simulink model "MassflowModel"  (R2020b)
settings: Solver=VariableStepAuto  StartTime=0.0  StopTime=55.357742309570312  RelTol=1e-3  AbsTol=1e-3
values from neighbouring files (symbols this model uses):
  coil_specific_heat_transfer = 20    [LoadDataForParameterEstimation.m]
  coil_voltage = 20    [LoadDataForParameterEstimation.m]
libraries: fl_lib x13, nesl_utility x10, SimscapeFluids_lib x1, SignalEditorBlockLib x1
(part 1 of 3)
settings Model: OrderedModelArguments=off  Creator=gam19  LastModifiedBy=gianandrea
settings SolverCC: AutoScaleAbsTol=off
settings DataIOCC: SaveOutput=off  SignalLogging=off  DSMLogging=off  SaveTime=off  ReturnWorkspaceOutputs=off  OutputTimes='[]'  ReturnWorkspaceOutputsName=SDOSimTest_Log
settings DebuggingCC: SymbolicDimsDataTypeCodeGenerationDiagnostic=none
settings SFSimCC: CustomCodeUndefinedFunction=UseInterfaceOnly
settings SimscapeCC: SimscapeLogType=all  SimscapeLogSimulationStatistics=on  SimscapeLogDataHistory=10000

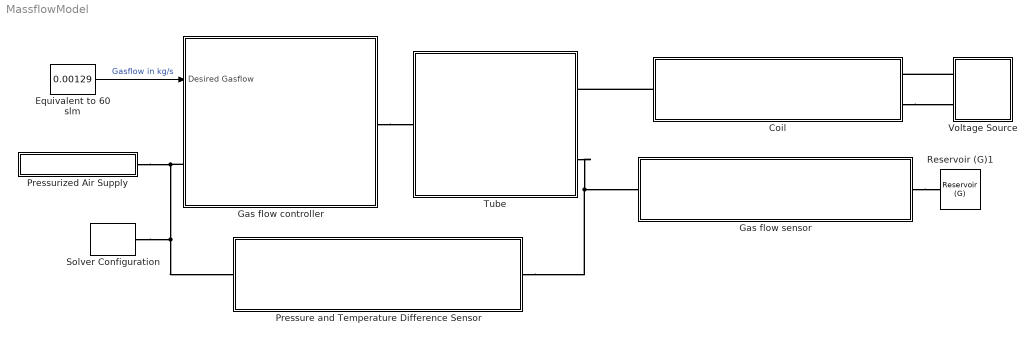
== system MassflowModel ==
  Coil : Subsystem
  Equivalent to 60 slm : Constant  Value=0.00129
  Gas flow controller : Subsystem
  Gas flow sensor : Subsystem
  Pressure and Temperature Difference Sensor : Subsystem
  Pressurized Air Supply : Subsystem
  Reservoir (G)1 : fl_lib/Gas/Elements/Reservoir (G)  pressure_spec=foundation.enum.pressure_spec.atmospheric  reservoir_pressure=0.101325 MPa  reservoir_temperature=300 K  area_A=0.01 m^2
      settings: SourceProductBaseCode=SS
  Solver Configuration : nesl_utility/Solver Configuration  PhysicalDomain=network_engine_domain  SubClassName=solver  LeftPortType=input  RightPortType=generic  Tones=[]  Harmonics=[]  SimulateNoise=off  Profile=off  UseLocalSampling=off  EnableSwitchedLinearOptims=on  FrequencyDomain=off  UseCCode=off  RelTol=0.001  AbsTol=1e-06  MinStep=1e-09  ToWorkspace=off  RevertToSquareIcSolve=off  NumHomotopyIterations=100  PhasorMode=off  PhasorModeNumHarmonics=1  DoDC=off  ResidualTolerance=1e-09  UseLocalSolver=off  LocalSolverChoice=NE_BACKWARD_EULER_ADVANCER  LocalSolverSampleTime=0.001  DoFixedCost=off  MaxNonlinIter=3  MaxModeIter=2  ComputeImpulses=off  ImpulseIterations=2  LinearAlgebra=auto  EquationFormulation=NE_TIME_EF  DelaysMemoryBudget=1024  AutomaticFiltering=on  FilteringTimeConstant=0.001  PartitionStorageMethod=AS_NEEDED  PartitionMemoryBudget=1024  PartitionMethod=ROBUST
  Tube : Subsystem
  Voltage Source : Subsystem
  wires:
  Equivalent to 60 slm/1 -> Gas flow controller/1(Desired Gasflow)  "Gasflow in kg/s"
  connections:
  Pressurized Air Supply/RConn1 -- Pressure and Temperature Difference Sensor/LConn1 -- Solver Configuration/RConn1 -- Gas flow controller/LConn1
  Gas flow controller/RConn1 -- Tube/LConn1
  Coil/LConn1 -- Tube/RConn1
  Tube/RConn2 -- Pressure and Temperature Difference Sensor/RConn1 -- Gas flow sensor/LConn1
  Gas flow sensor/RConn1 -- Reservoir (G)1/LConn1
  Voltage Source/LConn1 -- Coil/RConn1
  Coil/RConn2 -- Voltage Source/LConn2

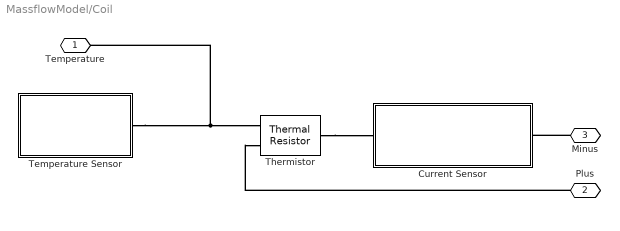
== system MassflowModel/Coil ==
  Current Sensor : Subsystem
  Temperature Sensor : Subsystem
  Thermistor : fl_lib/Electrical/Electrical Elements/Thermal Resistor  R0=9.5 Ohm  T0=298.15 K  alpha=50e-8 1/K  tc=coil_thermal_timeconstant s  K_d=0.0001 W/K  T_specify=off  T_priority=High  T=300 K  T_nominal_specify=off  T_nominal_unit=K  T_nominal_value=1
      settings: SourceProductBaseCode=SS  InternalSimscapePortConfiguration="{\"Bottom\":[],\"Left\":[{\"id\":\"H\",\"label\":\"H\",\"type\":\"foundation.thermal.thermal\"},{\"id\":\"p\",\"label\":\"+\",\"type\":\"foundation.electrical.electrical\"}],\"Right\":[{\"id\":\"n\",\"label\":\"-\",\"type\":\"foundation.electrical.electrical\"}],\"Top\":[]}"
  Temperature : PMIOPort  Side=Left
  Plus : PMIOPort  Port=2  Side=Right
  Minus : PMIOPort  Port=3  Side=Right
  connections:
  Plus/RConn1 -- Thermistor/LConn2
  Temperature/RConn1 -- Temperature Sensor/RConn1 -- Thermistor/LConn1
  Thermistor/RConn1 -- Current Sensor/LConn1
  Minus/RConn1 -- Current Sensor/RConn1

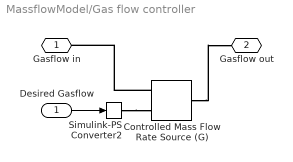
== system MassflowModel/Gas flow controller ==
  Desired Gasflow : Inport
  Controlled Mass Flow Rate Source (G) : fl_lib/Gas/Sources/Controlled Mass Flow Rate Source (G)  power_spec=foundation.enum.power_spec.isentropic  area_A=0.01 m^2  area_B=0.01 m^2
      settings: SourceProductBaseCode=SS  InternalSimscapePortConfiguration="{\"Bottom\":[],\"Left\":[{\"id\":\"A\",\"label\":\"A\",\"type\":\"foundation.gas.gas\"},{\"id\":\"M\",\"label\":\"M\",\"type\":\"input\"}],\"Right\":[{\"id\":\"B\",\"label\":\"B\",\"type\":\"foundation.gas.gas\"}],\"Top\":[]}"
  Simulink-PS Converter2 : nesl_utility/Simulink-PS Converter  PhysicalDomain=network_engine_domain  SubClassName=ps_input  LeftPortType=input  RightPortType=output  PseudoPeriodic=off  Frequencies=[]  NoiseDistribution=none  NoiseParameters=[]  Unit=kg/s  AffineConversion=off  FilteringAndDerivatives=provide  SimscapeFilterOrder=1  InputFilterTimeConstant=0.001  UdotUserProvided=0
  Gasflow in : PMIOPort  Side=Left
  Gasflow out : PMIOPort  Port=2  Side=Right
  wires:
  Desired Gasflow/1 -> Simulink-PS Converter2/1
  connections:
  Simulink-PS Converter2/RConn1 -- Controlled Mass Flow Rate Source (G)/LConn2
  Controlled Mass Flow Rate Source (G)/LConn1 -- Gasflow in/RConn1
  Controlled Mass Flow Rate Source (G)/RConn1 -- Gasflow out/RConn1

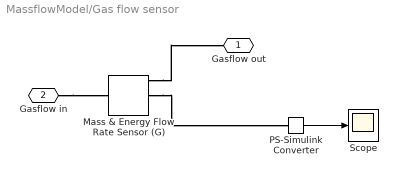
== system MassflowModel/Gas flow sensor ==
  Mass & Energy Flow Rate Sensor (G) : fl_lib/Gas/Sensors/Mass & Energy Flow Rate Sensor (G)
      settings: SourceProductBaseCode=SS  InternalSimscapePortConfiguration="{\"Bottom\":[],\"Left\":[{\"id\":\"A\",\"label\":\"A\",\"type\":\"foundation.gas.gas\"}],\"Right\":[{\"id\":\"B\",\"label\":\"B\",\"type\":\"foundation.gas.gas\"},{\"id\":\"M\",\"label\":\"M\",\"type\":\"output\"},{\"id\":\"PHI\",\"label\":\"Phi\",\"type\":\"output\"}],\"Top\":[]}"
  PS-Simulink Converter : nesl_utility/PS-Simulink Converter  PhysicalDomain=network_engine_domain  SubClassName=ps_output  LeftPortType=input  RightPortType=output  PseudoPeriodic=off  Frequencies=[]  Unit=inherit  AffineConversion=off
  Scope : Scope
  Gasflow out : PMIOPort  Side=Right
  Gasflow in : PMIOPort  Port=2  Side=Left
  wires:
  PS-Simulink Converter/1 -> Scope/1
  connections:
  Mass & Energy Flow Rate Sensor (G)/RConn2 -- PS-Simulink Converter/LConn1
  Mass & Energy Flow Rate Sensor (G)/RConn1 -- Gasflow out/RConn1
  Gasflow in/RConn1 -- Mass & Energy Flow Rate Sensor (G)/LConn1

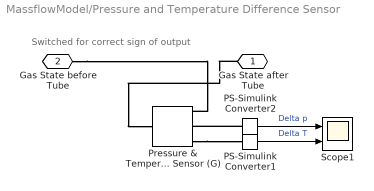
== system MassflowModel/Pressure and Temperature Difference Sensor ==
  note: Switched for correct sign of output
  PS-Simulink Converter1 : nesl_utility/PS-Simulink Converter  PhysicalDomain=network_engine_domain  SubClassName=ps_output  LeftPortType=input  RightPortType=output  PseudoPeriodic=off  Frequencies=[]  Unit=inherit  AffineConversion=off
  PS-Simulink Converter2 : nesl_utility/PS-Simulink Converter  PhysicalDomain=network_engine_domain  SubClassName=ps_output  LeftPortType=input  RightPortType=output  PseudoPeriodic=off  Frequencies=[]  Unit=Pa  AffineConversion=off
  Pressure & Temperature Sensor (G) : fl_lib/Gas/Sensors/Pressure & Temperature Sensor (G)
      settings: SourceProductBaseCode=SS  InternalSimscapePortConfiguration="{\"Bottom\":[],\"Left\":[{\"id\":\"A\",\"label\":\"A\",\"type\":\"foundation.gas.gas\"}],\"Right\":[{\"id\":\"B\",\"label\":\"B\",\"type\":\"foundation.gas.gas\"},{\"id\":\"P\",\"label\":\"P\",\"type\":\"output\"},{\"id\":\"T\",\"label\":\"T\",\"type\":\"output\"}],\"Top\":[]}"
  Scope1 : Scope  NumInputPorts=2
  Gas State after Tube : PMIOPort  Side=Right
  Gas State before Tube : PMIOPort  Port=2  Side=Left
  wires:
  PS-Simulink Converter1/1 -> Scope1/2  "Delta T"
  PS-Simulink Converter2/1 -> Scope1/1  "Delta p"
  connections:
  Pressure & Temperature Sensor (G)/RConn3 -- PS-Simulink Converter1/LConn1
  PS-Simulink Converter2/LConn1 -- Pressure & Temperature Sensor (G)/RConn2
  Gas State before Tube/RConn1 -- Pressure & Temperature Sensor (G)/RConn1
  Gas State after Tube/RConn1 -- Pressure & Temperature Sensor (G)/LConn1
